simulink model "gggg"  (R2016b)
settings: Solver=ode4  StartTime=0.0  StopTime=inf  FixedStep=0.002  RelTol=1e-3  EnableMultiTasking=on
undefined symbols (not defined in the file or in its folder): bit, Standard
libraries: slrtlib x8, slrtsoftinglib x8, dsparch4 x4
settings Model: SimulationMode=external  Creator=Administrator  LastModifiedBy=Administrator
settings SolverCC: EnableConcurrentExecution=on
settings DataIOCC: SaveFormat=StructureWithTime
settings OptimizationCC: BlockReduction=off  OptimizeBlockIOStorage=off  BufferReuse=off  GlobalBufferReuse=off  ExpressionFolding=off  LocalBlockOutputs=off
settings HardwareCC: ProdBitPerPointer=32  ProdBitPerSizeT=32  ProdBitPerPtrDiffT=32  ProdLargestAtomicFloat=None  ProdWordSize=32  ProdLongLongMode=on  ProdHWDeviceType=Generic->32-bit x86 compatible
settings RTWCC: SystemTargetFile=slrt.tlc  TemplateMakefile=slrt_default_tmf  Description=Simulink Real-Time  RTWCompilerOptimization=on

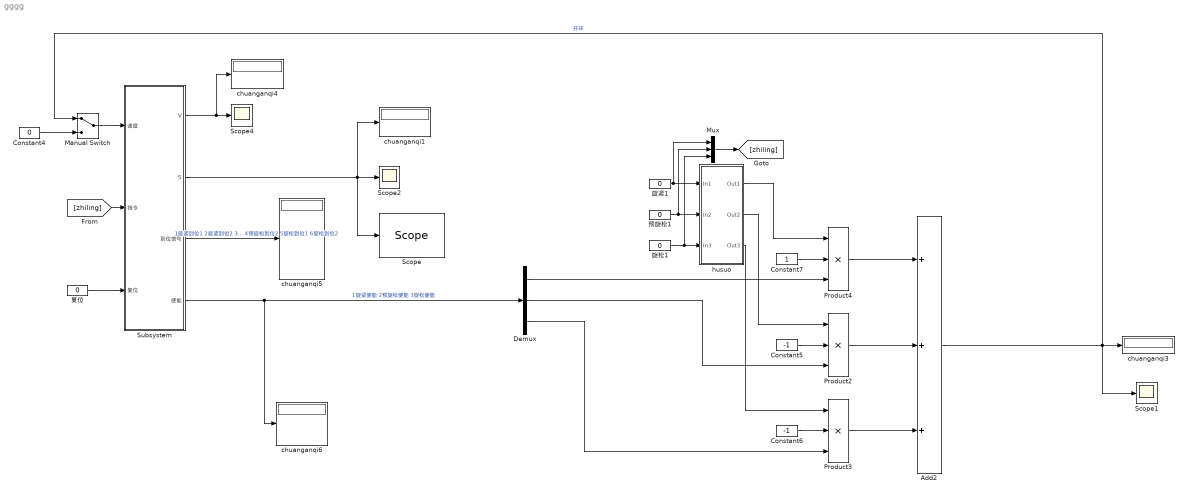
== system gggg ==
  Add2 : Sum  Inputs=+++
  Constant4 : Constant  Value=0
  Constant5 : Constant  Value=-1
  Constant6 : Constant  Value=-1
  Constant7 : Constant
  Demux : Demux  Outputs=3
  Manual Switch : ManualSwitch
  Mux : Mux  Inputs=3
  Product2 : Product  Inputs=3
  Product3 : Product  Inputs=3
  Product4 : Product  Inputs=3
  "Scope " : slrtlib/Displays and Logging/Scope   scopeno=1  scopetype=Target  autostart=on  viewmode=Graphical redraw  formatstr='%15.6f'  grid=on  ylimits=[0,0]  nosamples=250  noprepostsamples=0  interleave=1  triggermode=FreeRun  triggersignal=1  trigsignalfromport=off  triggerlevel=0.0  triggerslope=Either  triggerscope=1  triggersample=0  filename=data.dat  mode=Lazy  writesize=512  autorestart=off  dynamicfilemode=off  maxwritefilesize=512*1024^2
  Scope1 : Scope
  Scope2 : Scope
  Scope4 : Scope
  Subsystem : Subsystem
  chuanganqi{1,3..6} (5 alike) : Display
  husuo : Subsystem
  复位 : Constant  Value=0
      settings: OpenFcn=|
      | if get_param(gcb,'value')=='1',
      | set_param(gcb,'value','0');
      | else
      | set_param(gcb,'value','1');end
  旋松1 : Constant  Value=0
      settings: OpenFcn=|
      | if get_param(gcb,'value')=='1',
      | set_param(gcb,'value','0');
      | else
      | set_param(gcb,'value','1');end
  旋紧1 : Constant  Value=0
      settings: OpenFcn=|
      | if get_param(gcb,'value')=='1',
      | set_param(gcb,'value','0');
      | else
      | set_param(gcb,'value','1');end
  预旋松1 : Constant  Value=0
      settings: OpenFcn=|
      | if get_param(gcb,'value')=='1',
      | set_param(gcb,'value','0');
      | else
      | set_param(gcb,'value','1');end
  wires:
  Subsystem/2(S) -> chuanganqi1/1, "Scope "/1, Scope2/1
  Constant4/1 -> Manual Switch/2
  Manual Switch/1 -> Subsystem/1(速度)
  Subsystem/1(V) -> chuanganqi4/1, Scope4/1
  Subsystem/3(到位信号) -> chuanganqi5/1  "1旋紧到位1 2旋紧到位2 3预旋松到位1 4预旋松到位2 5旋松到位1 6旋松到位2"
  Subsystem/4(使能) -> chuanganqi6/1, Demux/1  "1旋紧使能 2预旋松使能 3旋松使能"
  Constant5/1 -> Product2/2
  Demux/2 -> Product2/3
  Constant6/1 -> Product3/2
  Demux/3 -> Product3/3
  Constant7/1 -> Product4/2
  Demux/1 -> Product4/3
  旋紧1/1 -> Mux/1, husuo/1(In1)
  预旋松1/1 -> Mux/2, husuo/2(In2)
  旋松1/1 -> Mux/3, husuo/3(In3)
  husuo/1(Out1) -> Product4/1
  husuo/2(Out2) -> Product2/1
  husuo/3(Out3) -> Product3/1
  Product4/1 -> Add2/1
  Product2/1 -> Add2/2
  Product3/1 -> Add2/3
  Add2/1 -> Manual Switch/1, Scope1/1, chuanganqi3/1  "开环"
  复位/1 -> Subsystem/3(复位)
  Mux/1 -> [zhiling]
  [zhiling] -> Subsystem/2(指令)

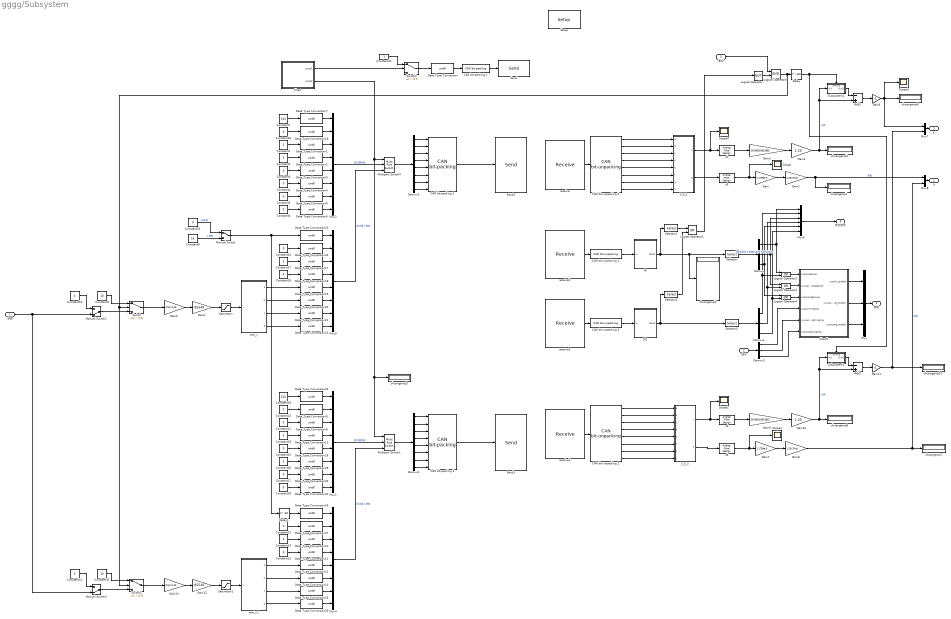
== system gggg/Subsystem ==
  速度 : Inport
  指令 : Inport  Port=2
  复位 : Inport  Port=3
  Add1 : Sum  Inputs=-+
  Add2 : Sum  Inputs=-+
  CAN bit-packing 1 : slrtlib/CAN/Utilities/CAN bit-packing   bitpatterns={[0:7]}
  CAN bit-packing 2 : slrtlib/CAN/Utilities/CAN bit-packing   bitpatterns={ [0:7] [8:15] [16:23] [24:31] [32:39] [40:47] [48:55] [56:63]}
  CAN bit-packing 3 : slrtlib/CAN/Utilities/CAN bit-packing   bitpatterns={ [0:7] [8:15] [16:23] [24:31] [32:39] [40:47] [48:55] [56:63]}
  CAN bit-unpacking 1 : slrtlib/CAN/Utilities/CAN bit-unpacking   bitpatterns={ [16:23] }  dtypes={ 'uint8'}
  CAN bit-unpacking 2 : slrtlib/CAN/Utilities/CAN bit-unpacking   bitpatterns={ [0:7] [8:15] [16:23] [24:31] [32:39] [40:47] [48:55] [56:63]}  dtypes={ 'uint8','uint8','uint8','uint8' ,'uint8','uint8','uint8','uint8'}
  CAN bit-unpacking 3 : slrtlib/CAN/Utilities/CAN bit-unpacking   bitpatterns={ [0:7] [8:15] [16:23] [24:31] [32:39] [40:47] [48:55] [56:63]}  dtypes={ 'uint8','uint8','uint8','uint8' ,'uint8','uint8','uint8','uint8'}
  CAN bit-unpacking 4 : slrtlib/CAN/Utilities/CAN bit-unpacking   bitpatterns={ [16:23] }  dtypes={ 'uint8'}
  Chart : Stateflow chart  TreatAsAtomicUnit=on
  Chart1 : Stateflow chart  TreatAsAtomicUnit=on
  Constant{1..2,11,14..15,17..19} (8 alike) : Constant  Value=3
  Constant{3..6,10,12..13,16,22..28} (15 alike) : Constant  Value=0
  Constant21 : Constant
  Constant29 : Constant  Value=134
  Constant31 : Constant  Value=10
  Constant7 : Constant  Value=134
  Constant8 : Constant  Value=15
  Constant9 : Constant  Value=10
  DI : MATLAB Function  TreatAsAtomicUnit=on
  DI1 : MATLAB Function  TreatAsAtomicUnit=on
  Data Type Conversion{,1..32} (33 alike) : DataTypeConversion  OutDataTypeStr=uint8
  Delay : Delay  DelayLength=250
  Delay1 : Delay  DelayLength=10
  Demux : Demux  Outputs=3
  Demux1 : Demux  Outputs=3
  Demux2 : Demux  Outputs=8
  Demux3 : Demux  Outputs=3
  Demux4 : Demux  Outputs=8
  Gain : Gain  Gain=1.1739e-5
  Gain1 : Gain  Gain=85546
  Gain10 : Gain  Gain=1.25
  Gain11 : Gain  Gain=-1
  Gain12 : Gain  Gain=85546
  Gain13 : Gain  Gain=(2*pi)/1.25
  Gain2 : Gain  Gain=1.25/(2*pi)
  Gain3 : Gain  Gain=59.9953/3931862
  Gain4 : Gain  Gain=1.25
  Gain5 : Gain  Gain=(2*pi)/1.25
  Gain6 : Gain  Gain=-1
  Gain7 : Gain  Gain=1.1739e-5
  Gain8 : Gain  Gain=1.25/(2*pi)
  Gain9 : Gain  Gain=59.9953/3931862
  Logical Operator : Logic  Operator=NOT  AllPortsSameDT=off  OutDataTypeStr=boolean
  Logical Operator{1..4} (4 alike) : Logic  Operator=OR  AllPortsSameDT=off  OutDataTypeStr=boolean
  Logical Operator6 : Logic  AllPortsSameDT=off  OutDataTypeStr=boolean
  Manual Switch : ManualSwitch
  Manual Switch1 : ManualSwitch  CurrentSetting=0
  Manual Switch3 : ManualSwitch  CurrentSetting=0
  Multiport Switch1 : MultiPortSwitch  DataPortOrder=Zero-based contiguous  Inputs=2
  Multiport Switch4 : MultiPortSwitch  DataPortOrder=Zero-based contiguous  Inputs=2
  Mux : Mux  Inputs=3
  Mux{1..4} (4 alike) : Mux  Inputs=8
  Mux6 : Mux  Inputs=6
  Mux7 : Mux  Inputs=2
  Mux8 : Mux  Inputs=2
  Saturation : Saturate  UpperLimit=2147483647  LowerLimit=-2147483647
  Saturation1 : Saturate  UpperLimit=2147483647  LowerLimit=-2147483647
  Scope{,1..4} (5 alike) : Scope
  Selector : Selector  IndexOptions=Index vector (dialog)  Indices=[1 2 3]  OutputSizes=1
  Selector1 : Selector  IndexOptions=Index vector (dialog)  Indices=1  OutputSizes=1
  Selector2 : Selector  IndexOptions=Index vector (dialog)  Indices=1  OutputSizes=1
  Selector3 : Selector  IndexOptions=Index vector (dialog)  Indices=[1 2 3]  OutputSizes=1
  Send : slrtsoftinglib/CAN-AC2-PCI SJA 1000/Send   board=1  canPort=CAN 2  range=Standard (11-bit)  ids=0  sizes=[8]  output=off  ts=-1  ididx=[0]
  Send1 : slrtsoftinglib/CAN-AC2-PCI SJA 1000/Send   board=1  canPort=CAN 2  range=Standard (11-bit)  ids=514  sizes=[8]  output=off  ts=-1  ididx=[2]
  Send2 : slrtsoftinglib/CAN-AC2-PCI SJA 1000/Send   board=1  canPort=CAN 2  range=Standard (11-bit)  ids=513  sizes=[8]  output=off  ts=-1  ididx=[1]
  "Setup " : slrtsoftinglib/CAN-AC2-PCI SJA 1000/Setup   board=1  can1bus=Highspeed (ISO 11898)  can1Baudrate=1 MBaud  can1UserBR=[1,1,4,3]  can2bus=Highspeed (ISO 11898)  can2Baudrate=500 kBaud  can2UserBR=[1,1,4,3]  init=[]  term=[]  bus_off_out=off  bus_off_rec=Off  ioBaseAddress=-1
  Subsystem1 : Subsystem
  Subsystem2 : Subsystem
  Switch : Switch  Criteria=u2 > Threshold  Threshold=0.5
  Switch1 : Switch  Criteria=u2 > Threshold  Threshold=0.5
  Switch2 : Switch  Criteria=u2 > Threshold  Threshold=0.5
  V_S_1 : MATLAB Function  TreatAsAtomicUnit=on
  V_S_2 : MATLAB Function  TreatAsAtomicUnit=on
  anti_v : MATLAB Function  TreatAsAtomicUnit=on
  anti_v1 : MATLAB Function  TreatAsAtomicUnit=on
  chuanganqi{1..4,6..8,10} (8 alike) : Display
  receive : slrtsoftinglib/CAN-AC2-PCI SJA 1000/Receive   board=1  canPort=CAN 2  range=Standard (11-bit)  ids=385  lengths=8  output=Data  inten=off  ts=-1  ididx=[0]
  receive1 : slrtsoftinglib/CAN-AC2-PCI SJA 1000/Receive   board=1  canPort=CAN 2  range=Standard (11-bit)  ids=386  lengths=8  output=Data  inten=off  ts=-1  ididx=[1]
  receive2 : slrtsoftinglib/CAN-AC2-PCI SJA 1000/Receive   board=1  canPort=CAN 2  range=Standard (11-bit)  ids=641  lengths=8  output=Data  inten=off  ts=-1  ididx=[2]
  receive3 : slrtsoftinglib/CAN-AC2-PCI SJA 1000/Receive   board=1  canPort=CAN 2  range=Standard (11-bit)  ids=642  lengths=8  output=Data  inten=off  ts=-1  ididx=[3]
  s{1,3..5} (4 alike) : dsparch4/Analog Filter Design  method=Butterworth  filttype=Lowpass  N=1  Wlo=10  Whi=80  Rp=2  Rs=40
  V : Outport
  S : Outport  Port=2
  到位信号 : Outport  Port=3
  使能 : Outport  Port=4
  wires:
  Data Type Conversion4/1 -> Mux2/6
  Constant6/1 -> Data Type Conversion6/1
  Constant2/1 -> Data Type Conversion2/1
  Constant16/1 -> Data Type Conversion16/1
  Data Type Conversion6/1 -> Mux2/8
  Data Type Conversion1/1 -> Mux2/3
  Data Type Conversion16/1 -> Mux2/2
  Constant7/1 -> Data Type Conversion7/1
  Constant1/1 -> Data Type Conversion1/1
  Data Type Conversion2/1 -> Mux2/4
  Constant5/1 -> Data Type Conversion5/1
  Data Type Conversion23/1 -> Mux3/1
  Data Type Conversion7/1 -> Mux2/1
  Data Type Conversion5/1 -> Mux2/7
  Constant4/1 -> Data Type Conversion4/1
  Data Type Conversion3/1 -> Mux2/5
  Data Type Conversion22/1 -> Mux3/8
  Constant18/1 -> Data Type Conversion18/1
  Demux2/3 -> CAN bit-packing 2/3
  Demux2/7 -> CAN bit-packing 2/7
  Data Type Conversion20/1 -> Mux3/6
  Data Type Conversion19/1 -> Mux3/5
  Constant24/1 -> Data Type Conversion24/1
  Demux2/8 -> CAN bit-packing 2/8
  Constant17/1 -> Data Type Conversion17/1
  Data Type Conversion17/1 -> Mux3/3
  Data Type Conversion24/1 -> Mux3/2
  Data Type Conversion21/1 -> Mux3/7
  Gain1/1 -> Saturation/1
  Data Type Conversion18/1 -> Mux3/4
  Demux2/1 -> CAN bit-packing 2/1
  Saturation/1 -> anti_v/1(v)
  Demux2/2 -> CAN bit-packing 2/2
  Demux2/4 -> CAN bit-packing 2/4
  Demux2/5 -> CAN bit-packing 2/5
  Demux2/6 -> CAN bit-packing 2/6
  Multiport Switch4/1 -> Demux2/1
  Mux3/1 -> Multiport Switch4/3  "驱动器上使能"
  CAN bit-packing 2/1 -> Send2/1
  Mux2/1 -> Multiport Switch4/2  "驱动器准备"
  Gain4/1 -> Add1/2, Subsystem2/1(In1), chuanganqi2/1  "位移"
  receive/1 -> CAN bit-unpacking 3/1
  CAN bit-unpacking 3/4 -> V_S_1/4(d)
  CAN bit-unpacking 3/2 -> V_S_1/2(b)
  Gain/1 -> Gain2/1
  CAN bit-unpacking 3/1 -> V_S_1/1(a)
  CAN bit-unpacking 3/3 -> V_S_1/3(c)
  s3/1 -> Scope/1, Gain/1
  V_S_1/1(V) -> Scope4/1, s1/1
  Gain3/1 -> Gain4/1
  Gain2/1 -> Mux8/1, chuanganqi1/1  "速度"
  Gain5/1 -> Gain1/1
  CAN bit-packing 1/1 -> Send/1
  Data Type Conversion/1 -> CAN bit-packing 1/1
  Switch2/1 -> Data Type Conversion/1
  Constant21/1 -> Switch2/1
  Constant3/1 -> Data Type Conversion3/1
  CAN bit-unpacking 3/5 -> V_S_1/5(e)
  CAN bit-unpacking 3/6 -> V_S_1/6(f)
  CAN bit-unpacking 3/7 -> V_S_1/7(g)
  CAN bit-unpacking 3/8 -> V_S_1/8(h)
  s1/1 -> Gain3/1
  Chart/1(route1) -> Switch2/2
  anti_v/4(d) -> Data Type Conversion22/1
  anti_v/2(b) -> Data Type Conversion20/1
  anti_v/1(a) -> Data Type Conversion19/1
  anti_v/3(c) -> Data Type Conversion21/1
  V_S_1/2(S) -> s3/1
  Manual Switch/1 -> Delay1/1, Data Type Conversion23/1
  Constant8/1 -> Manual Switch/2  "上使能"
  Constant23/1 -> Manual Switch/1  "去使能"
  receive2/1 -> CAN bit-unpacking 1/1
  CAN bit-unpacking 1/1 -> DI/1(a)
  DI/1(result) -> Selector/1, chuanganqi4/1, Selector1/1
  Constant10/1 -> Manual Switch1/1
  Manual Switch1/1 -> Switch/3
  Selector/1 -> Demux/1  "1旋紧到位 2预旋松到位 3旋松到位"
  Demux/1 -> Mux6/1, Logical Operator2/1
  Mux/1 -> 使能/1
  Subsystem2/1(Out1) -> Add1/1
  Logical Operator1/1 -> Logical Operator/1
  Add1/1 -> Gain6/1
  Gain6/1 -> Mux7/1, Scope3/1, chuanganqi6/1
  复位/1 -> Logical Operator6/1
  Switch/1 -> Gain5/1
  Constant9/1 -> Switch/1
  Logical Operator/1 -> Logical Operator6/2
  Delay/1 -> Subsystem1/Enable, Subsystem2/Enable
  Gain10/1 -> chuanganqi8/1, Subsystem1/1(In1), Add2/2  "位移"
  receive1/1 -> CAN bit-unpacking 2/1
  CAN bit-unpacking 2/4 -> V_S_2/4(d)
  CAN bit-unpacking 2/2 -> V_S_2/2(b)
  Gain7/1 -> Gain8/1
  CAN bit-unpacking 2/1 -> V_S_2/1(a)
  CAN bit-unpacking 2/3 -> V_S_2/3(c)
  s5/1 -> Gain7/1, Scope1/1
  V_S_2/1(V) -> s4/1, Scope2/1
  Gain9/1 -> Gain10/1
  Gain8/1 -> Mux8/2, chuanganqi7/1  "速度"
  CAN bit-unpacking 2/5 -> V_S_2/5(e)
  CAN bit-unpacking 2/6 -> V_S_2/6(f)
  CAN bit-unpacking 2/7 -> V_S_2/7(g)
  CAN bit-unpacking 2/8 -> V_S_2/8(h)
  s4/1 -> Gain9/1
  V_S_2/2(S) -> s5/1
  Gain11/1 -> Mux7/2, chuanganqi10/1
  Subsystem1/1(Out1) -> Add2/1
  Add2/1 -> Gain11/1
  receive3/1 -> CAN bit-unpacking 4/1
  CAN bit-unpacking 4/1 -> DI1/1(a)
  DI1/1(result) -> Selector3/1, Selector2/1
  Selector1/1 -> Logical Operator1/1
  Selector2/1 -> Logical Operator1/2
  Selector3/1 -> Demux1/1
  Demux/2 -> Mux6/3, Logical Operator3/1
  Demux/3 -> Logical Operator4/1, Mux6/5
  Demux1/1 -> Mux6/2, Logical Operator2/2
  Demux1/2 -> Mux6/4, Logical Operator3/2
  Demux1/3 -> Mux6/6, Logical Operator4/2
  Mux6/1 -> 到位信号/1
  Mux7/1 -> S/1
  Mux8/1 -> V/1
  指令/1 -> Demux3/1
  Logical Operator2/1 -> Chart1/1(xuanjindaowei)
  Logical Operator3/1 -> Chart1/2(yuxuansongdaowei)
  Logical Operator4/1 -> Chart1/3(xuansongdaowei)
  Chart1/1(xuanjin_enable) -> Mux/1
  Chart1/2(yuxuansong_enable) -> Mux/2
  Chart1/3(xuansong_enable) -> Mux/3
  Demux3/3 -> Chart1/6(xuansongmingling)
  Demux3/2 -> Chart1/5(yuxuansongmingling)
  Demux3/1 -> Chart1/4(xuanjinmingling)
  Data Type Conversion29/1 -> Mux1/6
  Constant28/1 -> Data Type Conversion31/1
  Constant19/1 -> Data Type Conversion13/1
  Constant13/1 -> Data Type Conversion9/1
  Data Type Conversion31/1 -> Mux1/8
  Data Type Conversion8/1 -> Mux1/3
  Data Type Conversion9/1 -> Mux1/2
  Constant29/1 -> Data Type Conversion32/1
  Constant11/1 -> Data Type Conversion8/1
  Data Type Conversion13/1 -> Mux1/4
  Constant27/1 -> Data Type Conversion30/1
  Data Type Conversion26/1 -> Mux4/1
  Data Type Conversion32/1 -> Mux1/1
  Data Type Conversion30/1 -> Mux1/7
  Constant26/1 -> Data Type Conversion29/1
  Data Type Conversion28/1 -> Mux1/5
  Data Type Conversion25/1 -> Mux4/8
  Constant15/1 -> Data Type Conversion11/1
  Demux4/3 -> CAN bit-packing 3/3
  Demux4/7 -> CAN bit-packing 3/7
  Data Type Conversion14/1 -> Mux4/6
  Data Type Conversion12/1 -> Mux4/5
  Constant22/1 -> Data Type Conversion27/1
  Demux4/8 -> CAN bit-packing 3/8
  Constant14/1 -> Data Type Conversion10/1
  Data Type Conversion10/1 -> Mux4/3
  Data Type Conversion27/1 -> Mux4/2
  Data Type Conversion15/1 -> Mux4/7
  Gain12/1 -> Saturation1/1
  Data Type Conversion11/1 -> Mux4/4
  Demux4/1 -> CAN bit-packing 3/1
  Saturation1/1 -> anti_v1/1(v)
  Demux4/2 -> CAN bit-packing 3/2
  Demux4/4 -> CAN bit-packing 3/4
  Demux4/5 -> CAN bit-packing 3/5
  Demux4/6 -> CAN bit-packing 3/6
  Multiport Switch1/1 -> Demux4/1
  Mux4/1 -> Multiport Switch1/3  "驱动器上使能"
  Mux1/1 -> Multiport Switch1/2  "驱动器准备"
  Gain13/1 -> Gain12/1
  Constant25/1 -> Data Type Conversion28/1
  anti_v1/4(d) -> Data Type Conversion25/1
  anti_v1/2(b) -> Data Type Conversion14/1
  anti_v1/1(a) -> Data Type Conversion12/1
  anti_v1/3(c) -> Data Type Conversion15/1
  Delay1/1 -> Data Type Conversion26/1
  Constant12/1 -> Manual Switch3/1
  Manual Switch3/1 -> Switch1/3
  Switch1/1 -> Gain13/1
  Constant31/1 -> Switch1/1
  Chart/2(route2) -> chuanganqi3/1, Multiport Switch1/1, Multiport Switch4/1
  速度/1 -> Manual Switch3/2, Manual Switch1/2
  Logical Operator6/1 -> Delay/1, Switch1/2, Switch/2
  CAN bit-packing 3/1 -> Send1/1

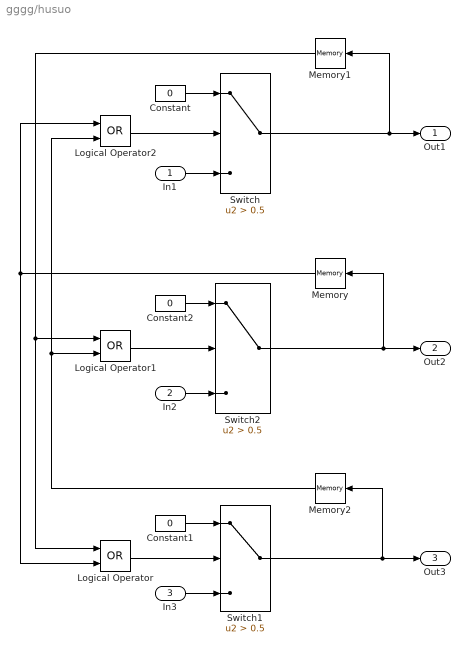
== system gggg/husuo ==
  In1 : Inport
  In2 : Inport  Port=2
  In3 : Inport  Port=3
  Constant : Constant  Value=0
  Constant1 : Constant  Value=0
  Constant2 : Constant  Value=0
  Logical Operator : Logic  Operator=OR  AllPortsSameDT=off  OutDataTypeStr=boolean
  Logical Operator1 : Logic  Operator=OR  AllPortsSameDT=off  OutDataTypeStr=boolean
  Logical Operator2 : Logic  Operator=OR  AllPortsSameDT=off  OutDataTypeStr=boolean
  Memory : Memory
  Memory1 : Memory
  Memory2 : Memory
  Switch : Switch  Criteria=u2 > Threshold  Threshold=0.5
  Switch1 : Switch  Criteria=u2 > Threshold  Threshold=0.5
  Switch2 : Switch  Criteria=u2 > Threshold  Threshold=0.5
  Out1 : Outport
  Out2 : Outport  Port=2
  Out3 : Outport  Port=3
  wires:
  Memory/1 -> Logical Operator2/1, Logical Operator/2
  Memory1/1 -> Logical Operator/1, Logical Operator1/1
  In1/1 -> Switch/3
  In2/1 -> Switch2/3
  Constant2/1 -> Switch2/1
  Switch/1 -> Memory1/1, Out1/1
  Constant/1 -> Switch/1
  Switch2/1 -> Memory/1, Out2/1
  In3/1 -> Switch1/3
  Constant1/1 -> Switch1/1
  Switch1/1 -> Memory2/1, Out3/1
  Logical Operator/1 -> Switch1/2
  Memory2/1 -> Logical Operator1/2, Logical Operator2/2
  Logical Operator1/1 -> Switch2/2
  Logical Operator2/1 -> Switch/2

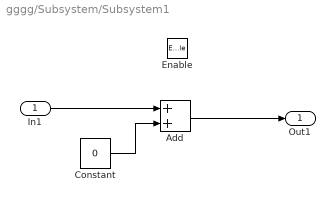
== system gggg/Subsystem/Subsystem1 ==
  In1 : Inport
  Enable : EnablePort
  Add : Sum
  Constant : Constant  Value=0
  Out1 : Outport
  wires:
  Constant/1 -> Add/2
  Add/1 -> Out1/1
  In1/1 -> Add/1

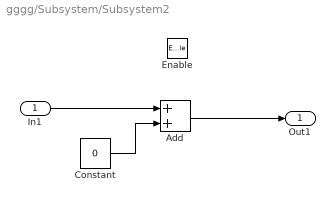
== system gggg/Subsystem/Subsystem2 ==
  In1 : Inport
  Enable : EnablePort
  Add : Sum
  Constant : Constant  Value=0
  Out1 : Outport
  wires:
  In1/1 -> Add/1
  Add/1 -> Out1/1
  Constant/1 -> Add/2

== matlab function gggg/Subsystem/anti_v ==
  data: v input; a output; b output; c output; d output
function [a, b, c, d]  = anti_velocity(v)
if v>=0
    BASE = '00000000000000000000000000000000';%一共32位
    Vbin = dec2bin(v);
    LVbin = length(Vbin);
    for i = 1:LVbin
        BASE(32-LVbin+i) = Vbin(i);
    end
    Vbin = BASE;
else
    BASE = '00000000000000000000000000000000';%一共32位
    V = 4294967295 + v + 1; %bin2dec('11111111111111111111111111111111')（一共32位）=4294967295
    Vbin = dec2bin(V);
    LVbin = length(Vbin);
    for i = 1:LVbin
        BASE(32-LVbin+i) = Vbin(i);
    end
    Vbin = BASE;
end
D = Vbin(1:8);
C = Vbin(9:16);
B = Vbin(17:24);
A = Vbin(25:32);
d = bin2dec(D);
c = bin2dec(C);
b = bin2dec(B);
a = bin2dec(A);
end

== matlab function gggg/Subsystem/V_S_1 ==
  data: a input; V output; b input; c input; d input; e input; f input; g input; h input; S output
function [V, S]  = conversion(a, b, c, d, e, f, g, h)
A = dec2bin(a);
B = dec2bin(b);
C = dec2bin(c);
D = dec2bin(d);
E = dec2bin(e);
F = dec2bin(f);
G = dec2bin(g);
H = dec2bin(h);

%% 速度
BASE = '00000000';
LA = length(A);
for i = 1:LA
    BASE(8-LA+i) = A(i);
end
A = BASE;

BASE = '00000000';
LB = length(B);
for i = 1:LB
    BASE(8-LB+i) = B(i);
end
B = BASE;

BASE = '00000000';
LC = length(C);
for i = 1:LC
    BASE(8-LC+i) = C(i);
end
C = BASE;

BASE = '00000000';
LD = length(D);
for i = 1:LD
    BASE(8-LD+i) = D(i);
end
D = BASE;

Vbin = [D, C, B, A];
R = bin2dec(Vbin);
if d < 128  %bin2dec('10000000')=128
    V = R;
else
    R = R-1;
    V = -(4294967295 - R); %bin2dec('11111111111111111111111111111111')（一共32位）=4294967295
end

%% 位移
BASE = '00000000';
LE = length(E);
for i = 1:LE
    BASE(8-LE+i) = E(i);
end
E = BASE;

BASE = '00000000';
LF = length(F);
for i = 1:LF
    BASE(8-LF+i) = F(i);
end
F = BASE;

BASE = '00000000';
LG = length(G);
for i = 1:LG
    BASE(8-LG+i) = G(i);
end
G = BASE;

BASE = '00000000';
LH = length(H);
for i = 1:LH
    BASE(8-LH+i) = H(i);
end
H = BASE;

Sbin = [H, G, F, E];
R = bin2dec(Sbin);
if h < 128  %bin2dec('10000000')=128
    S = R;
else
    R = R-1;
    S = -(4294967295 - R); %bin2dec('11111111111111111111111111111111')（一共32位）=4294967295
end

== matlab function gggg/Subsystem/V_S_2 ==
  data: a input; V output; b input; c input; d input; e input; f input; g input; h input; S output
function [V, S]  = conversion(a, b, c, d, e, f, g, h)
A = dec2bin(a);
B = dec2bin(b);
C = dec2bin(c);
D = dec2bin(d);
E = dec2bin(e);
F = dec2bin(f);
G = dec2bin(g);
H = dec2bin(h);

%% 速度
BASE = '00000000';
LA = length(A);
for i = 1:LA
    BASE(8-LA+i) = A(i);
end
A = BASE;

BASE = '00000000';
LB = length(B);
for i = 1:LB
    BASE(8-LB+i) = B(i);
end
B = BASE;

BASE = '00000000';
LC = length(C);
for i = 1:LC
    BASE(8-LC+i) = C(i);
end
C = BASE;

BASE = '00000000';
LD = length(D);
for i = 1:LD
    BASE(8-LD+i) = D(i);
end
D = BASE;

Vbin = [D, C, B, A];
R = bin2dec(Vbin);
if d < 128  %bin2dec('10000000')=128
    V = R;
else
    R = R-1;
    V = -(4294967295 - R); %bin2dec('11111111111111111111111111111111')（一共32位）=4294967295
end

%% 位移
BASE = '00000000';
LE = length(E);
for i = 1:LE
    BASE(8-LE+i) = E(i);
end
E = BASE;

BASE = '00000000';
LF = length(F);
for i = 1:LF
    BASE(8-LF+i) = F(i);
end
F = BASE;

BASE = '00000000';
LG = length(G);
for i = 1:LG
    BASE(8-LG+i) = G(i);
end
G = BASE;

BASE = '00000000';
LH = length(H);
for i = 1:LH
    BASE(8-LH+i) = H(i);
end
H = BASE;

Sbin = [H, G, F, E];
R = bin2dec(Sbin);
if h < 128  %bin2dec('10000000')=128
    S = R;
else
    R = R-1;
    S = -(4294967295 - R); %bin2dec('11111111111111111111111111111111')（一共32位）=4294967295
end

== stateflow chart gggg/Subsystem/Chart ==
  state route
    state on1
      en:
      route1=1;
      route2=0;
    state on3
      en:
      route1=0;
      route2=1;
    state on4
      en:
      route1=0;
      route2=2;
    (default) -> on1
    on1 -> on3 : after(10,tick)
    on3 -> on4 : after(10,tick)
  data: route1 output; route2 output

== matlab function gggg/Subsystem/DI ==
  data: a input; result output
function result  = conversion(a)
A = dec2bin(a);

BASE = '00000000';
LA = length(A);
for i = 1:LA
    BASE(8-LA+i) = A(i);
end
A = BASE;

a1 = bin2dec(A(1));
a2 = bin2dec(A(2));
a3 = bin2dec(A(3));
a4 = bin2dec(A(4));
a5 = bin2dec(A(5));
a6 = bin2dec(A(6));
a7 = bin2dec(A(7));
a8 = bin2dec(A(8));

result = [a8 a7 a6 a5 a4 a3 a2 a1];

== stateflow chart gggg/Subsystem/Chart1 ==
  state enable
    state enable1 [parallel]
      settings: executionOrder=1
      state on1
        en:
        xuanjin_enable=1;
      state on3
        en:
        xuanjin_enable=0;
      state on4
        en:
        xuanjin_enable=1;
      (default) -> enable.enable1.on1
      enable.enable1.on4 -> enable.enable1.on1 : [xuanjindaowei==0]
      enable.enable1.on1 -> enable.enable1.on3 : [xuanjindaowei==1]
      enable.enable1.on3 -> enable.enable1.on4 : [yuxuansongmingling==1||xuansongmingling==1]
    state enable2 [parallel]
      settings: executionOrder=2
      state on1
        en:
        yuxuansong_enable=1;
      state on3
        en:
        yuxuansong_enable=0;
      state on4
        en:
        yuxuansong_enable=1;
      (default) -> enable.enable2.on1
      enable.enable2.on4 -> enable.enable2.on1 : [yuxuansongdaowei==0]
      enable.enable2.on1 -> enable.enable2.on3 : [yuxuansongdaowei==1]
      enable.enable2.on3 -> enable.enable2.on4 : [xuansongmingling==1||xuanjinmingling==1]
    state enable3 [parallel]
      settings: executionOrder=3
      state on1
        en:
        xuansong_enable=1;
      state on3
        en:
        xuansong_enable=0;
      state on4
        en:
        xuansong_enable=1;
      (default) -> enable.enable3.on1
      enable.enable3.on4 -> enable.enable3.on1 : [xuansongdaowei==0]
      enable.enable3.on1 -> enable.enable3.on3 : [xuansongdaowei==1]
      enable.enable3.on3 -> enable.enable3.on4 : [xuanjinmingling==1]
  data: xuanjindaowei input; yuxuansongdaowei input; xuansongdaowei input; xuanjin_enable output; yuxuansong_enable output; xuansong_enable output; xuanjinmingling input; yuxuansongmingling input; xuansongmingling input

== matlab function gggg/Subsystem/anti_v1 ==
  data: v input; a output; b output; c output; d output
function [a, b, c, d]  = anti_velocity(v)
if v>=0
    BASE = '00000000000000000000000000000000';%一共32位
    Vbin = dec2bin(v);
    LVbin = length(Vbin);
    for i = 1:LVbin
        BASE(32-LVbin+i) = Vbin(i);
    end
    Vbin = BASE;
else
    BASE = '00000000000000000000000000000000';%一共32位
    V = 4294967295 + v + 1; %bin2dec('11111111111111111111111111111111')（一共32位）=4294967295
    Vbin = dec2bin(V);
    LVbin = length(Vbin);
    for i = 1:LVbin
        BASE(32-LVbin+i) = Vbin(i);
    end
    Vbin = BASE;
end
D = Vbin(1:8);
C = Vbin(9:16);
B = Vbin(17:24);
A = Vbin(25:32);
d = bin2dec(D);
c = bin2dec(C);
b = bin2dec(B);
a = bin2dec(A);
end

== matlab function gggg/Subsystem/DI1 ==
  data: a input; result output
function result  = conversion(a)
A = dec2bin(a);

BASE = '00000000';
LA = length(A);
for i = 1:LA
    BASE(8-LA+i) = A(i);
end
A = BASE;

a1 = bin2dec(A(1));
a2 = bin2dec(A(2));
a3 = bin2dec(A(3));
a4 = bin2dec(A(4));
a5 = bin2dec(A(5));
a6 = bin2dec(A(6));
a7 = bin2dec(A(7));
a8 = bin2dec(A(8));

result = [a8 a7 a6 a5 a4 a3 a2 a1];
